simulink model "EPT"  (R2019b)
settings: Solver=FixedStepDiscrete  StartTime=0.0  StopTime=5  FixedStep=0.005  RelTol=1e-3  EnableMultiTasking=on
PreLoadFcn:
  | try, model_open; catch, disp('Error occurred while executing model pre-load callback: model_open.m'); disp('Please assure that the MATLAB working directory is set to the model directory before opening.'); end
InitFcn:
  | try, model_open; catch, end
undefined symbols (not defined in the file or in its folder): Bridge, GCM, H, ln, raptor_get_param_eval, raptor_get_safe_string, raptor_xcp_function
libraries: Raptor_lib x2810, simulink x374, hdlsllib x19
(part 5 of 45)

== system EPT/Foreground_TimeBase_5ms/Oil//Water//Pack Cooling System/Delay2 ==
  Condition : Inport
  TimeCount : Inport  Port=2
  Constant10 : Constant
  Constant11 : Constant  Value=0
  Constant8 : Constant  Value=0
  CycleTrigger : Subsystem
  Switch2 : Switch  Threshold=1
  Switch3 : Switch  Threshold=1
  Unit Delay1 : UnitDelay  SampleTime=-1  HasFrameUpgradeWarning=on
  Unit Delay3 : UnitDelay  SampleTime=-1  HasFrameUpgradeWarning=on
  Output : Outport  VectorParamsAs1DForOutWhenUnconnected=off
  wires:
  TimeCount/1 -> CycleTrigger/2(In2)
  Condition/1 -> Switch3/2
  Constant8/1 -> Switch2/1
  CycleTrigger/1(Trigger) -> Switch2/2, Unit Delay3/1
  Constant10/1 -> Switch2/3
  Switch3/1 -> CycleTrigger/1(In1)
  Switch2/1 -> Unit Delay1/1
  Constant11/1 -> Switch3/3
  Unit Delay1/1 -> Switch3/1
  Unit Delay3/1 -> Output/1

== system EPT/Foreground_TimeBase_5ms/Oil//Water//Pack Cooling System/Delay3 ==
  Condition : Inport
  TimeCount : Inport  Port=2
  Constant10 : Constant
  Constant11 : Constant  Value=0
  Constant8 : Constant  Value=0
  CycleTrigger : Subsystem
  Switch2 : Switch  Threshold=1
  Switch3 : Switch  Threshold=1
  Unit Delay1 : UnitDelay  SampleTime=-1  HasFrameUpgradeWarning=on
  Unit Delay3 : UnitDelay  SampleTime=-1  HasFrameUpgradeWarning=on
  Output : Outport  VectorParamsAs1DForOutWhenUnconnected=off
  wires:
  Unit Delay3/1 -> Output/1
  Unit Delay1/1 -> Switch3/1
  Constant11/1 -> Switch3/3
  Switch2/1 -> Unit Delay1/1
  Switch3/1 -> CycleTrigger/1(In1)
  Constant10/1 -> Switch2/3
  CycleTrigger/1(Trigger) -> Unit Delay3/1, Switch2/2
  Constant8/1 -> Switch2/1
  Condition/1 -> Switch3/2
  TimeCount/1 -> CycleTrigger/2(In2)

== system EPT/Foreground_TimeBase_5ms/Oil//Water//Pack Cooling System/Delay5 ==
  Condition : Inport
  TimeCount : Inport  Port=2
  Constant10 : Constant
  Constant11 : Constant  Value=0
  Constant8 : Constant  Value=0
  CycleTrigger : Subsystem
  Switch2 : Switch  Threshold=1
  Switch3 : Switch  Threshold=1
  Unit Delay1 : UnitDelay  SampleTime=-1  HasFrameUpgradeWarning=on
  Unit Delay3 : UnitDelay  SampleTime=-1  HasFrameUpgradeWarning=on
  Output : Outport  VectorParamsAs1DForOutWhenUnconnected=off
  wires:
  Unit Delay3/1 -> Output/1
  Unit Delay1/1 -> Switch3/1
  Constant11/1 -> Switch3/3
  Switch2/1 -> Unit Delay1/1
  Switch3/1 -> CycleTrigger/1(In1)
  Constant10/1 -> Switch2/3
  CycleTrigger/1(Trigger) -> Unit Delay3/1, Switch2/2
  Constant8/1 -> Switch2/1
  Condition/1 -> Switch3/2
  TimeCount/1 -> CycleTrigger/2(In2)

== system EPT/Foreground_TimeBase_5ms/Oil//Water//Pack Cooling System/Delay6 ==
  Condition : Inport
  TimeCount : Inport  Port=2
  Constant10 : Constant
  Constant11 : Constant  Value=0
  Constant8 : Constant  Value=0
  CycleTrigger : Subsystem
  Switch2 : Switch  Threshold=1
  Switch3 : Switch  Threshold=1
  Unit Delay1 : UnitDelay  SampleTime=-1  HasFrameUpgradeWarning=on
  Unit Delay3 : UnitDelay  SampleTime=-1  HasFrameUpgradeWarning=on
  Output : Outport  VectorParamsAs1DForOutWhenUnconnected=off
  wires:
  Unit Delay3/1 -> Output/1
  Unit Delay1/1 -> Switch3/1
  Constant11/1 -> Switch3/3
  Switch2/1 -> Unit Delay1/1
  Switch3/1 -> CycleTrigger/1(In1)
  Constant10/1 -> Switch2/3
  CycleTrigger/1(Trigger) -> Unit Delay3/1, Switch2/2
  Constant8/1 -> Switch2/1
  Condition/1 -> Switch3/2
  TimeCount/1 -> CycleTrigger/2(In2)

== system EPT/Foreground_TimeBase_5ms/Oil//Water//Pack Cooling System/Delay7 ==
  Condition : Inport
  TimeCount : Inport  Port=2
  Constant10 : Constant
  Constant11 : Constant  Value=0
  Constant8 : Constant  Value=0
  CycleTrigger : Subsystem
  Switch2 : Switch  Threshold=1
  Switch3 : Switch  Threshold=1
  Unit Delay1 : UnitDelay  SampleTime=-1  HasFrameUpgradeWarning=on
  Unit Delay3 : UnitDelay  SampleTime=-1  HasFrameUpgradeWarning=on
  Output : Outport  VectorParamsAs1DForOutWhenUnconnected=off
  wires:
  Unit Delay3/1 -> Output/1
  Unit Delay1/1 -> Switch3/1
  Constant11/1 -> Switch3/3
  Switch2/1 -> Unit Delay1/1
  Switch3/1 -> CycleTrigger/1(In1)
  Constant10/1 -> Switch2/3
  CycleTrigger/1(Trigger) -> Unit Delay3/1, Switch2/2
  Constant8/1 -> Switch2/1
  Condition/1 -> Switch3/2
  TimeCount/1 -> CycleTrigger/2(In2)

== system EPT/Foreground_TimeBase_5ms/Oil//Water//Pack Cooling System/Latch ==
  Latch : Inport
  Reset : Inport  Port=2
  Switch1 : Switch  Criteria=u2 > Threshold
  Switch3 : Switch  Criteria=u2 > Threshold
  Unit Delay1 : UnitDelay  SampleTime=-1  HasFrameUpgradeWarning=on
  Output : Outport  VectorParamsAs1DForOutWhenUnconnected=off
  wires:
  Unit Delay1/1 -> Switch1/3
  Switch3/1 -> Output/1, Unit Delay1/1
  Reset/1 -> Switch3/2
  Latch/1 -> Switch1/1, Switch1/2
  Switch1/1 -> Switch3/3

== system EPT/Foreground_TimeBase_5ms/Oil//Water//Pack Cooling System/Latch1 ==
  Latch : Inport
  Reset : Inport  Port=2
  Switch1 : Switch  Criteria=u2 > Threshold
  Switch3 : Switch  Criteria=u2 > Threshold
  Unit Delay1 : UnitDelay  SampleTime=-1  HasFrameUpgradeWarning=on
  Output : Outport  VectorParamsAs1DForOutWhenUnconnected=off
  wires:
  Unit Delay1/1 -> Switch1/3
  Switch3/1 -> Output/1, Unit Delay1/1
  Reset/1 -> Switch3/2
  Latch/1 -> Switch1/1, Switch1/2
  Switch1/1 -> Switch3/3

== system EPT/Foreground_TimeBase_5ms/Oil//Water//Pack Cooling System/Latch2 ==
  Latch : Inport
  Reset : Inport  Port=2
  Switch1 : Switch  Criteria=u2 > Threshold
  Switch3 : Switch  Criteria=u2 > Threshold
  Unit Delay1 : UnitDelay  SampleTime=-1  HasFrameUpgradeWarning=on
  Output : Outport  VectorParamsAs1DForOutWhenUnconnected=off
  wires:
  Switch1/1 -> Switch3/3
  Latch/1 -> Switch1/2, Switch1/1
  Reset/1 -> Switch3/2
  Switch3/1 -> Unit Delay1/1, Output/1
  Unit Delay1/1 -> Switch1/3

== system EPT/Foreground_TimeBase_5ms/Oil//Water//Pack Cooling System/OC ==
  WaterTemp : Inport
  PW : Inport  Port=2
  Constant : Constant  Value=100
  Product3 : Product
  Saturation Dynamic2 : simulink/Discontinuities/Saturation Dynamic  OutMin=[]  OutMax=[]  OutDataTypeStr=Inherit: Same as second input  OutDataType=fixdt(1, 16)  OutScaling=2^-10  DoSatur=off
  raptor_adjustment4 : Raptor_lib/Data Storage/raptor_adjustment  paramName='Cal_OilBumpIdleDuty_Low_Saturation'  nameSource=Parameter  initValue=0  dataType=double  storage=Calibration  calDispType=Number  calEnum={'False', 'True'}  calGain=1.0  calOffset=0.0  calMax=inf  calMin=-inf  calFormat='-1'  calUnit=''  calHelp=''  calAccess=1  calFunction=raptor_xcp_function(gcb)  calDispHeaders=off  calColHeaders={'Col1' 'Col2' 'Col3'}  calRowHeaders={'Row1' 'Row2' 'Row3'}
      settings: SourceProductName=Raptor
  raptor_table_1d6 : Raptor_lib/Table Lookup/raptor_table_1d  dataName='OilCoolingSystemTemp2Ft'  initValue=[0.5,1,1,1.2,2,5,10]  dataType=double  storage=Calibration  initValueX=[0,35,40,45,60,70,80]  dataTypeXY=double  storageXY=Calibration  calVisible=on  showTable=on  calGain=1.0  calOffset=0.0  calMax=Inf  calMin=-Inf  calFormat='-1'  calUnit=''  calHelp=''  showBreakpoint=on  dataNameX=[]  calGainX=1.0  calOffsetX=0.0  calMaxX=Inf  calMinX=-Inf  calFormatX='-1'  calUnitX=''  calHelpX=''  calAccess=1  calFunction=raptor_xcp_function(gcb)  measureEnable=off  mName=[raptor_get_param_eval(gcb,'dataName'), '_Output']
      settings: SourceProductName=Raptor
  Duty : Outport
  wires:
  WaterTemp/1 -> raptor_table_1d6/1
  Product3/1 -> Saturation Dynamic2/2
  raptor_table_1d6/1 -> Product3/1
  raptor_adjustment4/1 -> Saturation Dynamic2/3
  Constant/1 -> Saturation Dynamic2/1
  PW/1 -> Product3/2
  Saturation Dynamic2/1 -> Duty/1

== system EPT/Foreground_TimeBase_5ms/Oil//Water//Pack Cooling System/WC ==
  WaterTemp : Inport
  PW : Inport  Port=2
  Constant : Constant  Value=100
  Product3 : Product
  Saturation Dynamic2 : simulink/Discontinuities/Saturation Dynamic  OutMin=[]  OutMax=[]  OutDataTypeStr=Inherit: Same as second input  OutDataType=fixdt(1, 16)  OutScaling=2^-10  DoSatur=off
  raptor_adjustment4 : Raptor_lib/Data Storage/raptor_adjustment  paramName='Cal_WaterBumpIdleDuty_Low_Saturation'  nameSource=Parameter  initValue=0  dataType=double  storage=Calibration  calDispType=Number  calEnum={'False', 'True'}  calGain=1.0  calOffset=0.0  calMax=inf  calMin=-inf  calFormat='-1'  calUnit=''  calHelp=''  calAccess=1  calFunction=raptor_xcp_function(gcb)  calDispHeaders=off  calColHeaders={'Col1' 'Col2' 'Col3'}  calRowHeaders={'Row1' 'Row2' 'Row3'}
      settings: SourceProductName=Raptor
  raptor_table_1d4 : Raptor_lib/Table Lookup/raptor_table_1d  dataName='WaterCoolingSystemTemp2Ft'  initValue=[0.5,1,1,1.5,2,5,10]  dataType=double  storage=Calibration  initValueX=[0,35,40,45,50,55,60]  dataTypeXY=double  storageXY=Calibration  calVisible=on  showTable=on  calGain=1.0  calOffset=0.0  calMax=Inf  calMin=-Inf  calFormat='-1'  calUnit=''  calHelp=''  showBreakpoint=on  dataNameX=[]  calGainX=1.0  calOffsetX=0.0  calMaxX=Inf  calMinX=-Inf  calFormatX='-1'  calUnitX=''  calHelpX=''  calAccess=1  calFunction=raptor_xcp_function(gcb)  measureEnable=off  mName=[raptor_get_param_eval(gcb,'dataName'), '_Output']
      settings: SourceProductName=Raptor
  Duty : Outport
  wires:
  PW/1 -> Product3/2
  Constant/1 -> Saturation Dynamic2/1
  raptor_table_1d4/1 -> Product3/1
  Product3/1 -> Saturation Dynamic2/2
  WaterTemp/1 -> raptor_table_1d4/1
  Saturation Dynamic2/1 -> Duty/1
  raptor_adjustment4/1 -> Saturation Dynamic2/3

== system EPT/Foreground_TimeBase_5ms/System Initial/CAN_Setup_Related ==
  Init : Inport
  raptor_data_write26 : Raptor_lib/Data Storage/raptor_data_write  dataName='Flag_ECHS_CAN_Work'  dataShape=Scalar  idxSource=Input Port  idxRow=1  idxCol=1
      settings: SourceProductName=Raptor
  wires:
  Init/1 -> raptor_data_write26/1

== system EPT/Foreground_TimeBase_5ms/System Initial/Delay1 ==
  Condition : Inport
  TimeCount : Inport  Port=2
  Constant10 : Constant
  Constant11 : Constant  Value=0
  Constant8 : Constant  Value=0
  CycleTrigger : Subsystem
  Switch2 : Switch  Threshold=1
  Switch3 : Switch  Threshold=1
  Unit Delay1 : UnitDelay  SampleTime=-1  HasFrameUpgradeWarning=on
  Unit Delay3 : UnitDelay  SampleTime=-1  HasFrameUpgradeWarning=on
  Output : Outport  VectorParamsAs1DForOutWhenUnconnected=off
  wires:
  TimeCount/1 -> CycleTrigger/2(In2)
  Condition/1 -> Switch3/2
  Constant8/1 -> Switch2/1
  CycleTrigger/1(Trigger) -> Switch2/2, Unit Delay3/1
  Constant10/1 -> Switch2/3
  Switch3/1 -> CycleTrigger/1(In1)
  Switch2/1 -> Unit Delay1/1
  Constant11/1 -> Switch3/3
  Unit Delay1/1 -> Switch3/1
  Unit Delay3/1 -> Output/1

== system EPT/Foreground_TimeBase_5ms/System Initial/Mode_Related ==
  Init : Inport
  raptor_data_write16 : Raptor_lib/Data Storage/raptor_data_write  dataName='Flag_Drive_Mode'  dataShape=Scalar  idxSource=Input Port  idxRow=1  idxCol=1
      settings: SourceProductName=Raptor
  raptor_data_write17 : Raptor_lib/Data Storage/raptor_data_write  dataName='Flag_PreCHG'  dataShape=Scalar  idxSource=Input Port  idxRow=1  idxCol=1
      settings: SourceProductName=Raptor
  raptor_data_write18 : Raptor_lib/Data Storage/raptor_data_write  dataName='Flag_CHG_Mode'  dataShape=Scalar  idxSource=Input Port  idxRow=1  idxCol=1
      settings: SourceProductName=Raptor
  wires:
  Init/1 -> raptor_data_write18/1, raptor_data_write16/1, raptor_data_write17/1

== system EPT/Foreground_TimeBase_5ms/System Initial/Motor_Related ==
  Init : Inport
  Data Type Conversion3 : DataTypeConversion
  Data Type Conversion4 : DataTypeConversion
  raptor_data_write5 : Raptor_lib/Data Storage/raptor_data_write  dataName='ECHS_GEAR_CMD'  dataShape=Scalar  idxSource=Input Port  idxRow=1  idxCol=1
      settings: SourceProductName=Raptor
  raptor_data_write6 : Raptor_lib/Data Storage/raptor_data_write  dataName='ECHS_TRQ_CMD'  dataShape=Scalar  idxSource=Input Port  idxRow=1  idxCol=1
      settings: SourceProductName=Raptor
  wires:
  Data Type Conversion4/1 -> raptor_data_write6/1
  Init/1 -> Data Type Conversion4/1, Data Type Conversion3/1
  Data Type Conversion3/1 -> raptor_data_write5/1

== system EPT/Foreground_TimeBase_5ms/System Initial/PreCHG_Related ==
  Init : Inport
  raptor_data_write : Raptor_lib/Data Storage/raptor_data_write  dataName='Flag_PreCharge_Relay_On'  dataShape=Scalar  idxSource=Input Port  idxRow=1  idxCol=1
      settings: SourceProductName=Raptor
  raptor_data_write2 : Raptor_lib/Data Storage/raptor_data_write  dataName='Flag_HV_Drive_Relay_On'  dataShape=Scalar  idxSource=Input Port  idxRow=1  idxCol=1
      settings: SourceProductName=Raptor
  raptor_data_write6 : Raptor_lib/Data Storage/raptor_data_write  dataName='Flag_HV_Negative_Relay_On'  dataShape=Scalar  idxSource=Input Port  idxRow=1  idxCol=1
      settings: SourceProductName=Raptor
  wires:
  Init/1 -> raptor_data_write6/1, raptor_data_write2/1, raptor_data_write/1

== system EPT/Foreground_TimeBase_5ms/System Initial/Shutdown_Event_Related ==
  Trigger : TriggerPort  VariantControl=Variant  PortDimensions=1
  Constant : Constant  Value=0  OutDataTypeStr=boolean
  Relaybox_Related : Subsystem
  wires:
  Constant/1 -> Relaybox_Related/1(Init)

== system EPT/Foreground_TimeBase_5ms/System Initial/Shutdown_Event_Related1 ==
  Trigger : TriggerPort  VariantControl=Variant  PortDimensions=1
  Constant : Constant  Value=0  OutDataTypeStr=boolean
  raptor_data_write15 : Raptor_lib/Data Storage/raptor_data_write  dataName='Fault_Reset_Trigger'  dataShape=Scalar  idxSource=Input Port  idxRow=1  idxCol=1
      settings: SourceProductName=Raptor
  wires:
  Constant/1 -> raptor_data_write15/1

== system EPT/Foreground_TimeBase_5ms/System Initial/Shutdown_Event_Related2 ==
  Trigger : TriggerPort  VariantControl=Variant  PortDimensions=1
  Constant : Constant  Value=0  OutDataTypeStr=boolean
  raptor_data_write14 : Raptor_lib/Data Storage/raptor_data_write  dataName='Flag_PowerOff_Finished'  dataShape=Scalar  idxSource=Input Port  idxRow=1  idxCol=1
      settings: SourceProductName=Raptor
  raptor_data_write6 : Raptor_lib/Data Storage/raptor_data_write  dataName='Flag_Ign_Off'  dataShape=Scalar  idxSource=Input Port  idxRow=1  idxCol=1
      settings: SourceProductName=Raptor
  wires:
  Constant/1 -> raptor_data_write14/1, raptor_data_write6/1

== system EPT/Foreground_TimeBase_5ms/System Setup/Dyno_Test  ==
  Dyno Test : Subsystem
  raptor_data_def : Raptor_lib/Data Storage/raptor_data_def  dataName='Dyno_Test_TqPercent'  initValue=0  dataType=double  storage=Volatile (RAM)  calVisible=on  calType=Measurement  calDispType=Number  calEnum={'False', 'True'}  calGain=1.0  calOffset=0  calMin=-inf  calMax=inf  calFormat='-1'  calUnit=''  calHelp=''  calAccess=1  calFunction=raptor_xcp_function(gcb)  calDispHeaders=off  calColHeaders={'Col1' 'Col2' 'Col3'}  calRowHeaders={'Row1' 'Row2' 'Row3'}
      settings: SourceProductName=Raptor
  raptor_data_write1 : Raptor_lib/Data Storage/raptor_data_write  dataName='Dyno_Test_TqPercent'  dataShape=Scalar  idxSource=Input Port  idxRow=1  idxCol=1
      settings: SourceProductName=Raptor
  raptor_measurement1 : Raptor_lib/Data Storage/raptor_measurement  paramName='Tq_Inc_equ_Tq_Max'  nameSource=Parameter  calDispType=Number  calEnum={'False', 'True'}  calGain=1.0  calOffset=0.0  calMax=inf  calMin=-inf  calFormat='-1'  calUnit=''  calHelp=''  calAccess=1  calFunction=raptor_xcp_function(gcb)  calVisible=on
      settings: SourceProductName=Raptor
  wires:
  Dyno Test/2(Flag) -> raptor_measurement1/1
  Dyno Test/1(Command_Tq) -> raptor_data_write1/1

== system EPT/Foreground_TimeBase_5ms/System Setup/HV_Setup() ==
  note: Notes :
      | - If not Alarm,trigger into PreCHG status
      | - PreCHG is Finished ,System trigger into CHG Mode or Drive Mode
  note: Notes :
      | - 1. ECHS CMD N(11b) to setup the diving mode status ,and then CMD R(01b) or D(10b) to drive motor.
  note: Notes :
      | - CMD Drive_Mode(01b)
      | - CMD CHG_Mode(10b)
  Abs : Abs
  Bitwise Operator1 : simulink/Logic and Bit Operations/Bitwise Operator  logicop=AND  UseBitMask=on  BitMask=bin2dec('11')  BitMaskRealWorld=Stored Integer
  Bitwise Operator2 : simulink/Logic and Bit Operations/Bitwise Operator  logicop=AND  UseBitMask=on  BitMask=bin2dec('11')  BitMaskRealWorld=Stored Integer
  CHG_Mode : Subsystem  TreatAsAtomicUnit=on
  Compare To Constant1 : simulink/Logic and Bit Operations/Compare To Constant  relop===  const=2  OutDataTypeStr=boolean
  Compare To Constant4 : simulink/Logic and Bit Operations/Compare To Constant  relop===  const=1  OutDataTypeStr=boolean
  Constant : Constant  Value=0
  Constant1 : Constant  Value=0  OutDataTypeStr=boolean
  Constant2 : Constant  Value=20
  Data Type Conversion{1..5} (5 alike) : DataTypeConversion
  Delay : Subsystem
  Drive_Mode : Subsystem  TreatAsAtomicUnit=on
  HV Setup Flow Chart : Stateflow chart  BlockKeywords=__PRM__SERIALIZED__DATA__:Stateflow Chart,Stateflow Diagram  TreatAsAtomicUnit=on
  HV Setup Flow Chart2 : Stateflow chart  Commented=on  BlockKeywords=__PRM__SERIALIZED__DATA__:Stateflow Chart,Stateflow Diagram  TreatAsAtomicUnit=on
  Latch : Subsystem
  Logical Operator : Logic  Operator=OR  AllPortsSameDT=off  OutDataTypeStr=boolean
  Logical Operator1 : Logic  AllPortsSameDT=off  OutDataTypeStr=boolean
  Logical Operator2 : Logic  Operator=OR  AllPortsSameDT=off  OutDataTypeStr=boolean
  Logical Operator3 : Logic  AllPortsSameDT=off  OutDataTypeStr=boolean
  NOT : Logic  Operator=NOT  IconShape=distinctive  AllPortsSameDT=off  OutDataTypeStr=boolean
  NOT1 : Logic  Operator=NOT  IconShape=distinctive  AllPortsSameDT=off  OutDataTypeStr=boolean
  PreCharge_Arbitration : Subsystem
  Subsystem : Subsystem  Commented=on
  raptor_adjustment1 : Raptor_lib/Data Storage/raptor_adjustment  paramName='Res'  nameSource=Parameter  initValue=30  dataType=double  storage=Calibration  calDispType=Number  calEnum={'False', 'True'}  calGain=1.0  calOffset=0.0  calMax=inf  calMin=-inf  calFormat='-1'  calUnit=''  calHelp=''  calAccess=1  calFunction=raptor_xcp_function(gcb)  calDispHeaders=off  calColHeaders={'Col1' 'Col2' 'Col3'}  calRowHeaders={'Row1' 'Row2' 'Row3'}
      settings: SourceProductName=Raptor
  raptor_adjustment2 : Raptor_lib/Data Storage/raptor_adjustment  paramName='Cal_HV_Off_Current_Adjustment'  nameSource=Parameter  initValue=50  dataType=Inherit via back propagation  storage=Calibration  calDispType=Number  calEnum={'False', 'True'}  calGain=1.0  calOffset=0.0  calMax=inf  calMin=-inf  calFormat='-1'  calUnit=''  calHelp=''  calAccess=1  calFunction=raptor_xcp_function(gcb)  calDispHeaders=off  calColHeaders={'Col1' 'Col2' 'Col3'}  calRowHeaders={'Row1' 'Row2' 'Row3'}
      settings: SourceProductName=Raptor
  raptor_adjustment3 : Raptor_lib/Data Storage/raptor_adjustment  paramName='Cap'  nameSource=Parameter  initValue=10000  dataType=double  storage=Calibration  calDispType=Number  calEnum={'False', 'True'}  calGain=1.0  calOffset=0.0  calMax=inf  calMin=-inf  calFormat='-1'  calUnit=''  calHelp=''  calAccess=1  calFunction=raptor_xcp_function(gcb)  calDispHeaders=off  calColHeaders={'Col1' 'Col2' 'Col3'}  calRowHeaders={'Row1' 'Row2' 'Row3'}
      settings: SourceProductName=Raptor
  raptor_data_def1 : Raptor_lib/Data Storage/raptor_data_def  dataName='Flag_Drive_Mode'  initValue=0  dataType=boolean  storage=Calibration  calVisible=on  calType=Measurement  calDispType=Number  calEnum={'False', 'True'}  calGain=1.0  calOffset=0  calMin=-inf  calMax=inf  calFormat='-1'  calUnit=''  calHelp=''  calAccess=1  calFunction=raptor_xcp_function(gcb)  calDispHeaders=off  calColHeaders={'Col1' 'Col2' 'Col3'}  calRowHeaders={'Row1' 'Row2' 'Row3'}
      settings: SourceProductName=Raptor
  raptor_data_def10 : Raptor_lib/Data Storage/raptor_data_def  dataName='HV_Setup_State'  initValue=0  dataType=uint8  storage=Volatile (RAM)  calVisible=on  calType=Measurement  calDispType=Number  calEnum={'False', 'True'}  calGain=1.0  calOffset=0  calMin=-inf  calMax=inf  calFormat='-1'  calUnit=''  calHelp=''  calAccess=1  calFunction=raptor_xcp_function(gcb)  calDispHeaders=off  calColHeaders={'Col1' 'Col2' 'Col3'}  calRowHeaders={'Row1' 'Row2' 'Row3'}
      settings: SourceProductName=Raptor
  raptor_data_def2 : Raptor_lib/Data Storage/raptor_data_def  dataName='HV_Off_State'  initValue=0  dataType=uint8  storage=Volatile (RAM)  calVisible=on  calType=Measurement  calDispType=Number  calEnum={'False', 'True'}  calGain=1.0  calOffset=0  calMin=-inf  calMax=inf  calFormat='-1'  calUnit=''  calHelp=''  calAccess=1  calFunction=raptor_xcp_function(gcb)  calDispHeaders=off  calColHeaders={'Col1' 'Col2' 'Col3'}  calRowHeaders={'Row1' 'Row2' 'Row3'}
      settings: SourceProductName=Raptor
  raptor_data_def27 : Raptor_lib/Data Storage/raptor_data_def  dataName='Flag_CHG_Mode'  initValue=0  dataType=boolean  storage=Calibration  calVisible=on  calType=Measurement  calDispType=Number  calEnum={'False', 'True'}  calGain=1.0  calOffset=0  calMin=-inf  calMax=inf  calFormat='-1'  calUnit=''  calHelp=''  calAccess=1  calFunction=raptor_xcp_function(gcb)  calDispHeaders=off  calColHeaders={'Col1' 'Col2' 'Col3'}  calRowHeaders={'Row1' 'Row2' 'Row3'}
      settings: SourceProductName=Raptor
  raptor_data_def4 : Raptor_lib/Data Storage/raptor_data_def  dataName='Flag_PreCHG'  initValue=0  dataType=boolean  storage=Volatile (RAM)  calVisible=on  calType=Measurement  calDispType=Number  calEnum={'False', 'True'}  calGain=1.0  calOffset=0  calMin=-inf  calMax=inf  calFormat='-1'  calUnit=''  calHelp=''  calAccess=1  calFunction=raptor_xcp_function(gcb)  calDispHeaders=off  calColHeaders={'Col1' 'Col2' 'Col3'}  calRowHeaders={'Row1' 'Row2' 'Row3'}
      settings: SourceProductName=Raptor
  raptor_data_read : Raptor_lib/Data Storage/raptor_data_read  dataName='Flag_PreCharge_Relay_On'  dataShape=Scalar  idxSource=Input  idxRow=1  idxCol=1
      settings: SourceProductName=Raptor
  raptor_data_read15 : Raptor_lib/Data Storage/raptor_data_read  dataName='EPT_BPOBU_VOLT'  dataShape=Scalar  idxSource=Input  idxRow=1  idxCol=1
      settings: SourceProductName=Raptor
  raptor_data_read16 : Raptor_lib/Data Storage/raptor_data_read  dataName='EPT_BPOBU_CURR'  dataShape=Scalar  idxSource=Input  idxRow=1  idxCol=1
      settings: SourceProductName=Raptor
  raptor_data_read17 : Raptor_lib/Data Storage/raptor_data_read  dataName='EPT_HV_BUS_VOLT'  dataShape=Scalar  idxSource=Input  idxRow=1  idxCol=1
      settings: SourceProductName=Raptor
  raptor_data_read2 : Raptor_lib/Data Storage/raptor_data_read  dataName='Flag_PreCharge_Relay_On'  dataShape=Scalar  idxSource=Input  idxRow=1  idxCol=1
      settings: SourceProductName=Raptor
  raptor_data_read5 : Raptor_lib/Data Storage/raptor_data_read  dataName='EPT_EW_STA'  dataShape=Scalar  idxSource=Input  idxRow=1  idxCol=1
      settings: SourceProductName=Raptor
  raptor_data_read6 : Raptor_lib/Data Storage/raptor_data_read  dataName='HV_Off'  dataShape=Scalar  idxSource=Input  idxRow=1  idxCol=1
      settings: SourceProductName=Raptor
  raptor_data_read7 : Raptor_lib/Data Storage/raptor_data_read  dataName='ECHS_VEH_MODE_REQ'  dataShape=Scalar  idxSource=Input  idxRow=1  idxCol=1
      settings: SourceProductName=Raptor
  raptor_data_write : Raptor_lib/Data Storage/raptor_data_write  dataName='Flag_PreCharge_Relay_On'  dataShape=Scalar  idxSource=Input Port  idxRow=1  idxCol=1
      settings: SourceProductName=Raptor
  raptor_data_write1 : Raptor_lib/Data Storage/raptor_data_write  dataName='Flag_Drive_Mode'  dataShape=Scalar  idxSource=Input Port  idxRow=1  idxCol=1
      settings: SourceProductName=Raptor
  raptor_data_write2 : Raptor_lib/Data Storage/raptor_data_write  dataName='Flag_CHG_Mode'  dataShape=Scalar  idxSource=Input Port  idxRow=1  idxCol=1
      settings: SourceProductName=Raptor
  raptor_data_write3 : Raptor_lib/Data Storage/raptor_data_write  dataName='Flag_PreCHG'  dataShape=Scalar  idxSource=Input Port  idxRow=1  idxCol=1
      settings: SourceProductName=Raptor
  raptor_data_write4 : Raptor_lib/Data Storage/raptor_data_write  dataName='Flag_HV_Drive_Relay_On'  dataShape=Scalar  idxSource=Input Port  idxRow=1  idxCol=1
      settings: SourceProductName=Raptor
  raptor_data_write5 : Raptor_lib/Data Storage/raptor_data_write  dataName='Flag_HV_Negative_Relay_On'  dataShape=Scalar  idxSource=Input Port  idxRow=1  idxCol=1
      settings: SourceProductName=Raptor
  raptor_data_write6 : Raptor_lib/Data Storage/raptor_data_write  dataName='HV_Setup_State'  dataShape=Scalar  idxSource=Input Port  idxRow=1  idxCol=1
      settings: SourceProductName=Raptor
  raptor_data_write7 : Raptor_lib/Data Storage/raptor_data_write  dataName='HV_Off_State'  dataShape=Scalar  idxSource=Input Port  idxRow=1  idxCol=1
      settings: SourceProductName=Raptor
  raptor_measurement : Raptor_lib/Data Storage/raptor_measurement  paramName='Meas_HV_On'  nameSource=Parameter  calDispType=Number  calEnum={'False', 'True'}  calGain=1.0  calOffset=0.0  calMax=inf  calMin=-inf  calFormat='-1'  calUnit=''  calHelp=''  calAccess=1  calFunction=raptor_xcp_function(gcb)  calVisible=on
      settings: SourceProductName=Raptor
  raptor_override : Raptor_lib/Data Storage/raptor_override  paramName='Cal_Flag_Drive_Mode'  nameSource=Parameter  measurement=None  calDispType=Number  calEnum={'False', 'True'}  calGain=1.0  calOffset=0.0  calMax=inf  calMin=-inf  calFormat='-1'  calUnit=''  calHelp=''  calAccess=1  calFunction=[raptor_xcp_function(gcb) '|' raptor_get_param_eval(gcb, 'paramName') '_Override']
      settings: SourceProductName=Raptor
  raptor_override1 : Raptor_lib/Data Storage/raptor_override  paramName='Cal_Flag_CHG_Mode'  nameSource=Parameter  measurement=None  calDispType=Number  calEnum={'False', 'True'}  calGain=1.0  calOffset=0.0  calMax=inf  calMin=-inf  calFormat='-1'  calUnit=''  calHelp=''  calAccess=1  calFunction=[raptor_xcp_function(gcb) '|' raptor_get_param_eval(gcb, 'paramName') '_Override']
      settings: SourceProductName=Raptor
  raptor_override2 : Raptor_lib/Data Storage/raptor_override  paramName='Cal_Flag_PreCHG_Mode'  nameSource=Parameter  measurement=None  calDispType=Number  calEnum={'False', 'True'}  calGain=1.0  calOffset=0.0  calMax=inf  calMin=-inf  calFormat='-1'  calUnit=''  calHelp=''  calAccess=1  calFunction=[raptor_xcp_function(gcb) '|' raptor_get_param_eval(gcb, 'paramName') '_Override']
      settings: SourceProductName=Raptor
  wires:
  Compare To Constant4/1 -> raptor_override/1
  raptor_data_read7/1 -> Bitwise Operator2/1, Bitwise Operator1/1
  Bitwise Operator1/1 -> Compare To Constant4/1
  Bitwise Operator2/1 -> Compare To Constant1/1
  Compare To Constant1/1 -> raptor_override1/1
  raptor_override1/1 -> [Chg_Mode], raptor_data_write2/1
  raptor_override/1 -> [Drive_Mode], raptor_data_write1/1
  raptor_override2/1 -> raptor_data_write3/1
  Constant1/1 -> raptor_override2/1
  PreCharge_Arbitration/1(PreCHG_Arbitration) -> Logical Operator1/2
  raptor_data_read/1 -> Logical Operator1/1
  Data Type Conversion1/1 -> raptor_data_write/1
  Data Type Conversion4/1 -> raptor_data_write4/1
  HV Setup Flow Chart/3(HV_Drive_Relay) -> Data Type Conversion4/1
  raptor_data_read16/1 -> Abs/1
  Latch/1(Output) -> HV Setup Flow Chart/2(PreCHG_Arbitration_Successful)
  raptor_data_read17/1 -> PreCharge_Arbitration/2(HV_Bus_Voltage)
  NOT/1 -> Latch/2(Reset)
  raptor_data_read15/1 -> PreCharge_Arbitration/1(HV_BPOBU_Voltage)
  raptor_adjustment1/1 -> PreCharge_Arbitration/3(Res)
  HV Setup Flow Chart/1(PreCHG_Relay) -> Data Type Conversion1/1
  Logical Operator1/1 -> Delay/1(Condition)
  Constant2/1 -> Delay/2(TimeCount)
  Delay/1(Output) -> Latch/1(Latch)
  raptor_adjustment2/1 -> HV Setup Flow Chart/4(HV_Current_Adjustment)
  raptor_adjustment3/1 -> PreCharge_Arbitration/4(Cap)
  raptor_data_read2/1 -> NOT/1
  HV Setup Flow Chart/2(HV_Negative_Relay) -> Data Type Conversion2/1
  Data Type Conversion2/1 -> raptor_data_write5/1
  HV Setup Flow Chart/5(HV_Setup_State) -> Data Type Conversion3/1
  Data Type Conversion3/1 -> raptor_data_write6/1
  HV Setup Flow Chart/4(HV_Off_State) -> Data Type Conversion5/1
  Data Type Conversion5/1 -> raptor_data_write7/1
  Abs/1 -> HV Setup Flow Chart/3(HV_Current)
  Constant/1 -> HV Setup Flow Chart/5(Emergency_HV_Off)
  [Drive_Mode] -> Logical Operator/1
  [Chg_Mode] -> Logical Operator/2
  Logical Operator3/1 -> raptor_measurement/1, HV Setup Flow Chart/1(HV_On)
  Logical Operator/1 -> Logical Operator3/1
  raptor_data_read5/1 -> Logical Operator2/1
  raptor_data_read6/1 -> Logical Operator2/2
  Logical Operator2/1 -> NOT1/1
  NOT1/1 -> Logical Operator3/2

== system EPT/Foreground_TimeBase_5ms/System Setup/Unit_Setup() ==
  Compare To Constant : simulink/Logic and Bit Operations/Compare To Constant  relop===  const=3  OutDataTypeStr=boolean
  Compare To Constant1 : simulink/Logic and Bit Operations/Compare To Constant  relop=>=  const=1  OutDataTypeStr=boolean
  Constant : Constant  OutDataTypeStr=boolean
  Data Type Conversion : DataTypeConversion
  Delay : Subsystem
  Delay1 : Subsystem
  Delay2 : Subsystem
  Delay3 : Subsystem
  Delay4 : Subsystem
  ECHS_CAN_Work : Subsystem  TreatAsAtomicUnit=on
  Logical Operator : Logic  AllPortsSameDT=off  OutDataTypeStr=boolean
  NOT3 : Logic  Operator=NOT  IconShape=distinctive  AllPortsSameDT=off  OutDataTypeStr=boolean
  Relay_DCDC_12V_Off : Subsystem  TreatAsAtomicUnit=on
  Relay_DCDC_12V_On : Subsystem  TreatAsAtomicUnit=on
  "Relay_HV_Body_Off " : Subsystem  TreatAsAtomicUnit=on
  "Relay_HV_Body_On " : Subsystem  TreatAsAtomicUnit=on
  raptor_adjustment1 : Raptor_lib/Data Storage/raptor_adjustment  paramName='Delay_DCDC12_On'  nameSource=Parameter  initValue=100  dataType=Inherit via back propagation  storage=Calibration  calDispType=Number  calEnum={'False', 'True'}  calGain=1.0  calOffset=0.0  calMax=inf  calMin=-inf  calFormat='-1'  calUnit=''  calHelp=''  calAccess=1  calFunction=raptor_xcp_function(gcb)  calDispHeaders=off  calColHeaders={'Col1' 'Col2' 'Col3'}  calRowHeaders={'Row1' 'Row2' 'Row3'}
      settings: SourceProductName=Raptor
  raptor_adjustment2 : Raptor_lib/Data Storage/raptor_adjustment  paramName='Delay_DCDC12V_Off'  nameSource=Parameter  initValue=100  dataType=Inherit via back propagation  storage=Calibration  calDispType=Number  calEnum={'False', 'True'}  calGain=1.0  calOffset=0.0  calMax=inf  calMin=-inf  calFormat='-1'  calUnit=''  calHelp=''  calAccess=1  calFunction=raptor_xcp_function(gcb)  calDispHeaders=off  calColHeaders={'Col1' 'Col2' 'Col3'}  calRowHeaders={'Row1' 'Row2' 'Row3'}
      settings: SourceProductName=Raptor
  raptor_adjustment4 : Raptor_lib/Data Storage/raptor_adjustment  paramName='Cal_Delay_ECHS_CAN_Controller_PowerOn'  nameSource=Parameter  initValue=100  dataType=Inherit via back propagation  storage=Calibration  calDispType=Number  calEnum={'False', 'True'}  calGain=1.0  calOffset=0.0  calMax=inf  calMin=-inf  calFormat='-1'  calUnit=''  calHelp=''  calAccess=1  calFunction=raptor_xcp_function(gcb)  calDispHeaders=off  calColHeaders={'Col1' 'Col2' 'Col3'}  calRowHeaders={'Row1' 'Row2' 'Row3'}
      settings: SourceProductName=Raptor
  raptor_adjustment5 : Raptor_lib/Data Storage/raptor_adjustment  paramName='Delay_Relay_HV_Body_On'  nameSource=Parameter  initValue=100  dataType=Inherit via back propagation  storage=Calibration  calDispType=Number  calEnum={'False', 'True'}  calGain=1.0  calOffset=0.0  calMax=inf  calMin=-inf  calFormat='-1'  calUnit=''  calHelp=''  calAccess=1  calFunction=raptor_xcp_function(gcb)  calDispHeaders=off  calColHeaders={'Col1' 'Col2' 'Col3'}  calRowHeaders={'Row1' 'Row2' 'Row3'}
      settings: SourceProductName=Raptor
  raptor_adjustment6 : Raptor_lib/Data Storage/raptor_adjustment  paramName='Delay_Relay_HV_Body_Off'  nameSource=Parameter  initValue=100  dataType=Inherit via back propagation  storage=Calibration  calDispType=Number  calEnum={'False', 'True'}  calGain=1.0  calOffset=0.0  calMax=inf  calMin=-inf  calFormat='-1'  calUnit=''  calHelp=''  calAccess=1  calFunction=raptor_xcp_function(gcb)  calDispHeaders=off  calColHeaders={'Col1' 'Col2' 'Col3'}  calRowHeaders={'Row1' 'Row2' 'Row3'}
      settings: SourceProductName=Raptor
  raptor_data_read1 : Raptor_lib/Data Storage/raptor_data_read  dataName='EPT_EW_STA'  dataShape=Scalar  idxSource=Input  idxRow=1  idxCol=1
      settings: SourceProductName=Raptor
  raptor_data_read2 : Raptor_lib/Data Storage/raptor_data_read  dataName='HV_Off_State'  dataShape=Scalar  idxSource=Input  idxRow=1  idxCol=1
      settings: SourceProductName=Raptor
  raptor_data_read4 : Raptor_lib/Data Storage/raptor_data_read  dataName='Flag_SystemStart'  dataShape=Scalar  idxSource=Input  idxRow=1  idxCol=1
      settings: SourceProductName=Raptor
  raptor_data_read8 : Raptor_lib/Data Storage/raptor_data_read  dataName='HV_Setup_State'  dataShape=Scalar  idxSource=Input  idxRow=1  idxCol=1
      settings: SourceProductName=Raptor
  raptor_data_write : Raptor_lib/Data Storage/raptor_data_write  dataName='Relay_BMS_OBU'  dataShape=Scalar  idxSource=Input Port  idxRow=1  idxCol=1
      settings: SourceProductName=Raptor
  raptor_data_write1 : Raptor_lib/Data Storage/raptor_data_write  dataName='Relay_BMS_SWU'  dataShape=Scalar  idxSource=Input Port  idxRow=1  idxCol=1
      settings: SourceProductName=Raptor
  raptor_data_write11 : Raptor_lib/Data Storage/raptor_data_write  dataName='EPT_READY'  dataShape=Scalar  idxSource=Input Port  idxRow=1  idxCol=1
      settings: SourceProductName=Raptor
  wires:
  raptor_adjustment4/1 -> Delay/2(TimeCount)
  Delay3/1(Output) -> Relay_DCDC_12V_On/Trigger
  raptor_adjustment1/1 -> Delay3/2(TimeCount)
  raptor_adjustment2/1 -> Delay4/2(TimeCount)
  Delay/1(Output) -> ECHS_CAN_Work/Trigger
  Delay4/1(Output) -> Relay_DCDC_12V_Off/Trigger
  raptor_data_read4/1 -> Logical Operator/2
  Delay2/1(Output) -> "Relay_HV_Body_Off "/Trigger
  raptor_adjustment6/1 -> Delay2/2(TimeCount)
  raptor_adjustment5/1 -> Delay1/2(TimeCount)
  Delay1/1(Output) -> "Relay_HV_Body_On "/Trigger
  raptor_data_read8/1 -> Compare To Constant/1
  Logical Operator/1 -> Data Type Conversion/1
  Data Type Conversion/1 -> raptor_data_write11/1
  raptor_data_read1/1 -> NOT3/1
  NOT3/1 -> Logical Operator/1
  raptor_data_read2/1 -> Compare To Constant1/1
  Compare To Constant/1 -> Delay1/1(Condition), Delay3/1(Condition)
  Compare To Constant1/1 -> Delay2/1(Condition), Delay4/1(Condition)
  Constant/1 -> Delay/1(Condition), raptor_data_write1/1, raptor_data_write/1

== system EPT/I//O/Input/ADC_ChargerPlugInterface ==
  note: Standby
  note: Vehicle Detected
  note: Ready Charging
  note: No power
  note: Error
  Compare To Constant : simulink/Logic and Bit Operations/Compare To Constant  relop=>=  const=200  OutDataTypeStr=boolean
  Compare To Constant1 : simulink/Logic and Bit Operations/Compare To Constant  relop=<=  const=86  OutDataTypeStr=boolean
  Compare To Constant10 : simulink/Logic and Bit Operations/Compare To Constant  relop=<  const=8  OutDataTypeStr=boolean
  Compare To Constant11 : simulink/Logic and Bit Operations/Compare To Constant  relop=>  const=97  OutDataTypeStr=boolean
  Compare To Constant2 : simulink/Logic and Bit Operations/Compare To Constant  relop=>=  const=4.5  OutDataTypeStr=boolean
  Compare To Constant3 : simulink/Logic and Bit Operations/Compare To Constant  relop=>=  const=3.5  OutDataTypeStr=boolean
  Compare To Constant4 : simulink/Logic and Bit Operations/Compare To Constant  relop=<  const=4.5  OutDataTypeStr=boolean
  Compare To Constant5 : simulink/Logic and Bit Operations/Compare To Constant  relop=>=  const=2.5  OutDataTypeStr=boolean
  Compare To Constant6 : simulink/Logic and Bit Operations/Compare To Constant  relop=<  const=3.5  OutDataTypeStr=boolean
  Compare To Constant7 : simulink/Logic and Bit Operations/Compare To Constant  relop=>=  const=0.5  OutDataTypeStr=boolean
  Compare To Constant8 : simulink/Logic and Bit Operations/Compare To Constant  relop=<  const=1.5  OutDataTypeStr=boolean
  Compare To Constant9 : simulink/Logic and Bit Operations/Compare To Constant  relop=<  const=0.5  OutDataTypeStr=boolean
  Constant : Constant  Value=64
  Data Type Conversion : DataTypeConversion
  Data Type Conversion1 : DataTypeConversion
  Data Type Conversion2 : DataTypeConversion
  Delay1 : Subsystem
  Delay2 : Subsystem
  Delay3 : Subsystem
  Gain : Gain  Gain=5/4095
  Gain1 : Gain  Gain=100/4095
  Gain2 : Gain  Gain=100/4095
  Gain3 : Gain  Gain=0.6
  Gain4 : Gain  Gain=2.5
  Latch1 : Subsystem
  Latch2 : Subsystem
  Latch3 : Subsystem
  Logical Operator{,1..2,4..5} (5 alike) : Logic  AllPortsSameDT=off  OutDataTypeStr=boolean
  Logical Operator3 : Logic  Operator=OR  AllPortsSameDT=off  OutDataTypeStr=boolean
  Logical Operator6 : Logic  Operator=OR  AllPortsSameDT=off  OutDataTypeStr=boolean
  NOT{,1..3} (4 alike) : Logic  Operator=NOT  IconShape=distinctive  AllPortsSameDT=off  OutDataTypeStr=boolean
  Subtract : Sum  Inputs=+-
  Switch : Switch  Criteria=u2 > Threshold
  raptor_adjustment : Raptor_lib/Data Storage/raptor_adjustment  paramName='Cal_EVSE_STATUS_Delaytimes'  nameSource=Parameter  initValue=100  dataType=double  storage=Calibration  calDispType=Number  calEnum={'False', 'True'}  calGain=1.0  calOffset=0.0  calMax=inf  calMin=-inf  calFormat='-1'  calUnit=''  calHelp=''  calAccess=1  calFunction=raptor_xcp_function(gcb)  calDispHeaders=off  calColHeaders={'Col1' 'Col2' 'Col3'}  calRowHeaders={'Row1' 'Row2' 'Row3'}
      settings: SourceProductName=Raptor
  raptor_analog_in : Raptor_lib/Input & Output/raptor_analog_in  resourceValues=INPUT2|INPUT3|INPUT4|INPUT5|INPUT6|INPUT7|INPUT8|INPUT9|INPUT10|INPUT11|INPUT12|INPUT13|INPUT14|INPUT15|INPUT16|INPUT17|INPUT18|INPUT19|INPUT20|INPUT21|INPUT22|INPUT23|INPUT24|INPUT25|INPUT26|INPUT27|INPUT28|INPUT29|INPUT30|INPUT31|INPUT32|(None)  resource=INPUT4  pullUDValues=422k PD  pullUD=422k PD  rangeValues=0 - 5 V  range=0 - 5 V  filterrateValues=[]  filterrate='RAPTOR MASK DEFAULT'  resolutionValues=[]  resolution=[]
      settings: SourceProductName=Raptor
  raptor_analog_in1 : Raptor_lib/Input & Output/raptor_analog_in  resourceValues=INPUT2|INPUT3|INPUT4|INPUT5|INPUT6|INPUT7|INPUT8|INPUT9|INPUT10|INPUT11|INPUT12|INPUT13|INPUT14|INPUT15|INPUT16|INPUT17|INPUT18|INPUT19|INPUT20|INPUT21|INPUT22|INPUT23|INPUT24|INPUT25|INPUT26|INPUT27|INPUT28|INPUT29|INPUT30|INPUT31|INPUT32|(None)  resource=INPUT12  pullUDValues=422k PD  pullUD=422k PD  rangeValues=0 - 5 V  range=0 - 5 V  filterrateValues=[]  filterrate='RAPTOR MASK DEFAULT'  resolutionValues=[]  resolution=[]
      settings: SourceProductName=Raptor
  raptor_analog_in3 : Raptor_lib/Input & Output/raptor_analog_in  resourceValues=INPUT2|INPUT3|INPUT4|INPUT5|INPUT6|INPUT7|INPUT8|INPUT9|INPUT10|INPUT11|INPUT12|INPUT13|INPUT14|INPUT15|INPUT16|INPUT17|INPUT18|INPUT19|INPUT20|INPUT21|INPUT22|INPUT23|INPUT24|INPUT25|INPUT26|INPUT27|INPUT28|INPUT29|INPUT30|INPUT31|INPUT32|(None)  resource=INPUT30  pullUDValues=215k PD  pullUD=215k PD  rangeValues=0 - 5 V  range=0 - 5 V  filterrateValues=[]  filterrate='RAPTOR MASK DEFAULT'  resolutionValues=[]  resolution=[]
      settings: SourceProductName=Raptor
  raptor_analog_in4 : Raptor_lib/Input & Output/raptor_analog_in  resourceValues=INPUT2|INPUT3|INPUT4|INPUT5|INPUT6|INPUT7|INPUT8|INPUT9|INPUT10|INPUT11|INPUT12|INPUT13|INPUT14|INPUT15|INPUT16|INPUT17|INPUT18|INPUT19|INPUT20|INPUT21|INPUT22|INPUT23|INPUT24|INPUT25|INPUT26|INPUT27|INPUT28|INPUT29|INPUT30|INPUT31|INPUT32|(None)  resource=INPUT24  pullUDValues=56.7k PD  pullUD=56.7k PD  rangeValues=0 - 5 V  range=0 - 5 V  filterrateValues=[]  filterrate='RAPTOR MASK DEFAULT'  resolutionValues=[]  resolution=[]
      settings: SourceProductName=Raptor
  raptor_data_def : Raptor_lib/Data Storage/raptor_data_def  dataName='A18_EVSE_Status'  initValue=0  dataType=double  storage=Calibration  calVisible=on  calType=Measurement  calDispType=Number  calEnum={'False', 'True'}  calGain=1.0  calOffset=0  calMin=-inf  calMax=inf  calFormat='-1'  calUnit=''  calHelp=''  calAccess=1  calFunction=raptor_xcp_function(gcb)  calDispHeaders=off  calColHeaders={'Col1' 'Col2' 'Col3'}  calRowHeaders={'Row1' 'Row2' 'Row3'}
      settings: SourceProductName=Raptor
  raptor_data_def1 : Raptor_lib/Data Storage/raptor_data_def  dataName='A59_CHG_Level_Set'  initValue=0  dataType=double  storage=Calibration  calVisible=on  calType=Measurement  calDispType=Number  calEnum={'False', 'True'}  calGain=1.0  calOffset=0  calMin=-inf  calMax=inf  calFormat='-1'  calUnit=''  calHelp=''  calAccess=1  calFunction=raptor_xcp_function(gcb)  calDispHeaders=off  calColHeaders={'Col1' 'Col2' 'Col3'}  calRowHeaders={'Row1' 'Row2' 'Row3'}
      settings: SourceProductName=Raptor
  raptor_data_def2 : Raptor_lib/Data Storage/raptor_data_def  dataName='K82_EVSE_Capacity'  initValue=0  dataType=double  storage=Calibration  calVisible=on  calType=Measurement  calDispType=Number  calEnum={'False', 'True'}  calGain=1.0  calOffset=0  calMin=-inf  calMax=inf  calFormat='-1'  calUnit=''  calHelp=''  calAccess=1  calFunction=raptor_xcp_function(gcb)  calDispHeaders=off  calColHeaders={'Col1' 'Col2' 'Col3'}  calRowHeaders={'Row1' 'Row2' 'Row3'}
      settings: SourceProductName=Raptor
  raptor_data_def3 : Raptor_lib/Data Storage/raptor_data_def  dataName='K35_CHG_Request'  initValue=0  dataType=boolean  storage=Calibration  calVisible=on  calType=Measurement  calDispType=Number  calEnum={'False', 'True'}  calGain=1.0  calOffset=0  calMin=-inf  calMax=inf  calFormat='-1'  calUnit=''  calHelp=''  calAccess=1  calFunction=raptor_xcp_function(gcb)  calDispHeaders=off  calColHeaders={'Col1' 'Col2' 'Col3'}  calRowHeaders={'Row1' 'Row2' 'Row3'}
      settings: SourceProductName=Raptor
  raptor_data_def4 : Raptor_lib/Data Storage/raptor_data_def  dataName='EVSE_STATUS_A'  initValue=0  dataType=boolean  storage=Calibration  calVisible=on  calType=Measurement  calDispType=Number  calEnum={'False', 'True'}  calGain=1.0  calOffset=0  calMin=-inf  calMax=inf  calFormat='-1'  calUnit=''  calHelp=''  calAccess=1  calFunction=raptor_xcp_function(gcb)  calDispHeaders=off  calColHeaders={'Col1' 'Col2' 'Col3'}  calRowHeaders={'Row1' 'Row2' 'Row3'}
      settings: SourceProductName=Raptor
  raptor_data_def5 : Raptor_lib/Data Storage/raptor_data_def  dataName='EVSE_STATUS_B'  initValue=0  dataType=boolean  storage=Calibration  calVisible=on  calType=Measurement  calDispType=Number  calEnum={'False', 'True'}  calGain=1.0  calOffset=0  calMin=-inf  calMax=inf  calFormat='-1'  calUnit=''  calHelp=''  calAccess=1  calFunction=raptor_xcp_function(gcb)  calDispHeaders=off  calColHeaders={'Col1' 'Col2' 'Col3'}  calRowHeaders={'Row1' 'Row2' 'Row3'}
      settings: SourceProductName=Raptor
  raptor_data_def6 : Raptor_lib/Data Storage/raptor_data_def  dataName='EVSE_STATUS_C'  initValue=0  dataType=boolean  storage=Calibration  calVisible=on  calType=Measurement  calDispType=Number  calEnum={'False', 'True'}  calGain=1.0  calOffset=0  calMin=-inf  calMax=inf  calFormat='-1'  calUnit=''  calHelp=''  calAccess=1  calFunction=raptor_xcp_function(gcb)  calDispHeaders=off  calColHeaders={'Col1' 'Col2' 'Col3'}  calRowHeaders={'Row1' 'Row2' 'Row3'}
      settings: SourceProductName=Raptor
  raptor_data_def7 : Raptor_lib/Data Storage/raptor_data_def  dataName='EVSE_STATUS_E'  initValue=0  dataType=boolean  storage=Calibration  calVisible=on  calType=Measurement  calDispType=Number  calEnum={'False', 'True'}  calGain=1.0  calOffset=0  calMin=-inf  calMax=inf  calFormat='-1'  calUnit=''  calHelp=''  calAccess=1  calFunction=raptor_xcp_function(gcb)  calDispHeaders=off  calColHeaders={'Col1' 'Col2' 'Col3'}  calRowHeaders={'Row1' 'Row2' 'Row3'}
      settings: SourceProductName=Raptor
  raptor_data_def8 : Raptor_lib/Data Storage/raptor_data_def  dataName='EVSE_STATUS_F'  initValue=0  dataType=boolean  storage=Calibration  calVisible=on  calType=Measurement  calDispType=Number  calEnum={'False', 'True'}  calGain=1.0  calOffset=0  calMin=-inf  calMax=inf  calFormat='-1'  calUnit=''  calHelp=''  calAccess=1  calFunction=raptor_xcp_function(gcb)  calDispHeaders=off  calColHeaders={'Col1' 'Col2' 'Col3'}  calRowHeaders={'Row1' 'Row2' 'Row3'}
      settings: SourceProductName=Raptor
  raptor_data_write : Raptor_lib/Data Storage/raptor_data_write  dataName='A18_EVSE_Status'  dataShape=Scalar  idxSource=Input Port  idxRow=1  idxCol=1
      settings: SourceProductName=Raptor
  raptor_data_write1 : Raptor_lib/Data Storage/raptor_data_write  dataName='A59_CHG_Level_Set'  dataShape=Scalar  idxSource=Input Port  idxRow=1  idxCol=1
      settings: SourceProductName=Raptor
  raptor_data_write2 : Raptor_lib/Data Storage/raptor_data_write  dataName='K82_EVSE_Capacity'  dataShape=Scalar  idxSource=Input Port  idxRow=1  idxCol=1
      settings: SourceProductName=Raptor
  raptor_data_write3 : Raptor_lib/Data Storage/raptor_data_write  dataName='K35_CHG_Request'  dataShape=Scalar  idxSource=Input Port  idxRow=1  idxCol=1
      settings: SourceProductName=Raptor
  raptor_data_write5 : Raptor_lib/Data Storage/raptor_data_write  dataName='EVSE_STATUS_F'  dataShape=Scalar  idxSource=Input Port  idxRow=1  idxCol=1
      settings: SourceProductName=Raptor
  raptor_data_write6 : Raptor_lib/Data Storage/raptor_data_write  dataName='EVSE_STATUS_E'  dataShape=Scalar  idxSource=Input Port  idxRow=1  idxCol=1
      settings: SourceProductName=Raptor
  raptor_data_write7 : Raptor_lib/Data Storage/raptor_data_write  dataName='EVSE_STATUS_C'  dataShape=Scalar  idxSource=Input Port  idxRow=1  idxCol=1
      settings: SourceProductName=Raptor
  raptor_data_write8 : Raptor_lib/Data Storage/raptor_data_write  dataName='EVSE_STATUS_B'  dataShape=Scalar  idxSource=Input Port  idxRow=1  idxCol=1
      settings: SourceProductName=Raptor
  raptor_data_write9 : Raptor_lib/Data Storage/raptor_data_write  dataName='EVSE_STATUS_A'  dataShape=Scalar  idxSource=Input Port  idxRow=1  idxCol=1
      settings: SourceProductName=Raptor
  wires:
  raptor_analog_in/1 -> Gain/1
  raptor_analog_in1/1 -> Gain2/1
  raptor_analog_in3/1 -> Gain1/1
  raptor_analog_in4/1 -> Compare To Constant/1
  Gain/1 -> Data Type Conversion/1
  Compare To Constant/1 -> raptor_data_write3/1
  Gain1/1 -> Data Type Conversion2/1
  Gain2/1 -> Data Type Conversion1/1
  Data Type Conversion1/1 -> raptor_data_write1/1
  Switch/1 -> raptor_data_write2/1
  Compare To Constant1/1 -> Switch/2
  Gain3/1 -> Switch/1
  Subtract/1 -> Gain4/1
  Gain4/1 -> Switch/3
  Constant/1 -> Subtract/2
  Data Type Conversion2/1 -> Subtract/1, Gain3/1, Compare To Constant10/1, Compare To Constant11/1, Compare To Constant1/1
  Compare To Constant4/1 -> Logical Operator/1
  Compare To Constant3/1 -> Logical Operator/2
  Compare To Constant6/1 -> Logical Operator1/1
  Compare To Constant5/1 -> Logical Operator1/2
  Data Type Conversion/1 -> raptor_data_write/1, Compare To Constant2/1, Compare To Constant4/1, Compare To Constant3/1, Compare To Constant6/1, Compare To Constant5/1, Compare To Constant8/1, Compare To Constant7/1, Compare To Constant9/1
  Compare To Constant8/1 -> Logical Operator2/1
  Compare To Constant7/1 -> Logical Operator2/2
  Compare To Constant10/1 -> Logical Operator3/1
  Compare To Constant11/1 -> Logical Operator3/2
  Logical Operator2/1 -> Logical Operator4/1
  Compare To Constant9/1 -> Logical Operator5/1
  Logical Operator3/1 -> Logical Operator4/2, Logical Operator5/2, NOT3/1
  Logical Operator5/1 -> raptor_data_write5/1
  Logical Operator4/1 -> raptor_data_write6/1
  Delay1/1(Output) -> Latch1/2(Reset)
  Latch1/1(Output) -> raptor_data_write7/1
  Logical Operator/1 -> NOT1/1, Latch2/1(Latch)
  Delay2/1(Output) -> Latch2/2(Reset)
  Latch2/1(Output) -> raptor_data_write8/1
  NOT/1 -> Delay1/1(Condition)
  NOT1/1 -> Delay2/1(Condition)
  NOT2/1 -> Delay3/1(Condition)
  Delay3/1(Output) -> Latch3/2(Reset)
  Compare To Constant2/1 -> Latch3/1(Latch), NOT2/1
  Latch3/1(Output) -> raptor_data_write9/1
  raptor_adjustment/1 -> Delay3/2(TimeCount), Delay1/2(TimeCount), Delay2/2(TimeCount)
  Logical Operator1/1 -> Logical Operator6/1
  NOT3/1 -> Logical Operator6/2
  Logical Operator6/1 -> NOT/1, Latch1/1(Latch)
